simulink model "test_dc_motor_drive"  (R2025b)
settings: Solver=VariableStepAuto  StartTime=0.0  StopTime=8  RelTol=1e-3
StopFcn:
  | Simulink.sdi.view;
  | Simulink.sdi.loadView('view_dc_motor_drive.mldatx');
libraries: nesl_utility x5, fl_lib x4, ee_lib x1, arsenal x1, shareduavrstlib x1, simulink x1
settings Model: Creator=upattacini  LastModifiedBy=upattacini
settings SolverCC: DaesscMode=Robust  ZeroCrossAlgorithm=Adaptive  DecoupledContinuousIntegration=on  MinimalZcImpactIntegration=on
settings DataIOCC: SaveOutput=off  DSMLogging=off  SaveTime=off  ReturnWorkspaceOutputs=off

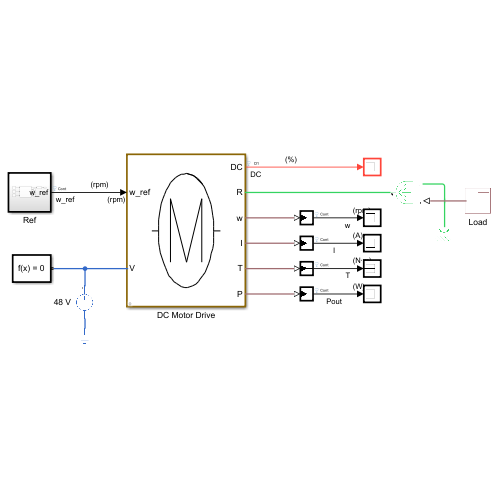
[thumbnail: Simulink's stored preview of the top-level diagram]
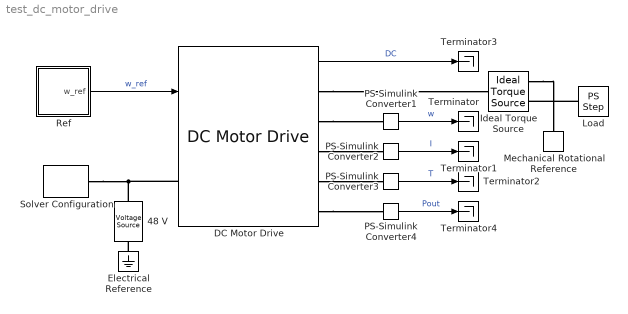
== system test_dc_motor_drive ==
  48 V : ee_lib/Sources/Voltage Source  dc_voltage=48 V  ac_voltage=0 V  ac_shift=0 rad  ac_frequency=60 Hz  noise_mode=ee.enum.sources.noise.Disabled  PSD=0 V^2/Hz  sample_time=1e-3 s  repeatability=ee.enum.sources.repeatability.NotRepeatable  user_seed=0  auto_seed=3499211588  i_specify=off  i_priority=None  i=0 A  i_nominal_specify=off  i_nominal_value=1  i_nominal_unit=A  v_specify=off  v_priority=None  v=0 V  v_nominal_specify=off  v_nominal_value=1  v_nominal_unit=V
  DC Motor Drive : arsenal/Simscape Components/Actuators/DC Motors/DC Motor Drive  R=0.58  L=0.0002  Kt=0.1564  T_bkpts=[0 0.774 1.564 2.71]  I_table=[0 4.95 10 17.325]  V_rated=48  GB_ratio=7.75  J=6.9927e-5  Kp=0.1  Ki=0.1  Ts=0.005  ff_bkpts=[0 60 120 180 240 310]  ff_table=[0 10 20 40 60 80]  V_max=100
  Electrical Reference : fl_lib/Electrical/Electrical Elements/Electrical Reference
  Ideal Torque Source : fl_lib/Mechanical/Mechanical Sources/Ideal Torque Source
  Load : fl_lib/Physical Signals/Sources/PS Step  step_time=4 s  initial_value=0 N*m  final_value=-1 N*m
  Mechanical Rotational Reference : fl_lib/Mechanical/Rotational Elements/Mechanical Rotational Reference
  PS-Simulink Converter1 : nesl_utility/PS-Simulink Converter  PhysicalDomain=network_engine_domain  SubClassName=ps_output  LeftPortType=input  RightPortType=output  PseudoPeriodic=off  Frequencies=[]  VectorFormat=inherit  Unit=rpm  AffineConversion=off
  PS-Simulink Converter2 : nesl_utility/PS-Simulink Converter  PhysicalDomain=network_engine_domain  SubClassName=ps_output  LeftPortType=input  RightPortType=output  PseudoPeriodic=off  Frequencies=[]  VectorFormat=inherit  Unit=A  AffineConversion=off
  PS-Simulink Converter3 : nesl_utility/PS-Simulink Converter  PhysicalDomain=network_engine_domain  SubClassName=ps_output  LeftPortType=input  RightPortType=output  PseudoPeriodic=off  Frequencies=[]  VectorFormat=inherit  Unit=N*m  AffineConversion=off
  PS-Simulink Converter4 : nesl_utility/PS-Simulink Converter  PhysicalDomain=network_engine_domain  SubClassName=ps_output  LeftPortType=input  RightPortType=output  PseudoPeriodic=off  Frequencies=[]  VectorFormat=inherit  Unit=W  AffineConversion=off
  Ref : Subsystem
  Solver Configuration : nesl_utility/Solver Configuration  PhysicalDomain=network_engine_domain  SubClassName=solver  LeftPortType=input  RightPortType=generic  Tones=[]  Harmonics=[]  SimulateNoise=off  Profile=off  UseLocalSampling=off  EnableSwitchedLinearOptims=on  FrequencyDomain=off  UseCCode=off  RelTol=0.001  AbsTol=0.001  MinStep=1e-09  ToWorkspace=off  RevertToSquareIcSolve=off  NumHomotopyIterations=100  PhasorMode=off  PhasorModeNumHarmonics=1  ConsistencySolver=NEWTON_XTOL_AFTER_FTOL  IndexReductionMethod=DerivativeReplacement  DoDC=off  ResidualTolerance=1e-09  ConsistencyTolSource=GLOBAL  ConsistencyAbsTol=0.001  ConsistencyRelTol=0.001  ConsistencyTolFactor=1  UseLocalSolver=off  LocalSolverChoice=NE_BACKWARD_EULER_ADVANCER  ResolveIndetEquations=on  FunctionEvalNumThread=1  LocalSolverSampleTime=0.001  DoFixedCost=off  MaxNonlinIter=3  MaxModeIter=2  ComputeImpulses=off  ImpulseIterations=2  LinearAlgebra=auto  LinearAlgebraNumThread=0  EquationFormulation=NE_TIME_EF  DelaysMemoryBudget=1024  AutomaticFiltering=on  FilteringTimeConstant=0.001  PartitionStorageMethod=AS_NEEDED  PartitionMemoryBudget=1024  PartitionMethod=ROBUST  MultibodyUseLocalSolver=off  MultibodyLocalSolverChoice=ODE1  MultibodyLocalSolverSampleTime=0.001
  Terminator{,1..4} (5 alike) : Terminator
  wires:
  Ref/1(w_ref) -> DC Motor Drive/1  "w_ref"
  PS-Simulink Converter2/1 -> Terminator1/1  "I"
  DC Motor Drive/1 -> Terminator3/1  "DC"
  PS-Simulink Converter1/1 -> Terminator/1  "w"
  PS-Simulink Converter3/1 -> Terminator2/1  "T"
  PS-Simulink Converter4/1 -> Terminator4/1  "Pout"
  connections:
  Electrical Reference/LConn1 -- 48 V/RConn1
  48 V/LConn1 -- Solver Configuration/RConn1 -- DC Motor Drive/LConn1
  DC Motor Drive/RConn3 -- PS-Simulink Converter2/LConn1
  DC Motor Drive/RConn2 -- PS-Simulink Converter1/LConn1
  DC Motor Drive/RConn4 -- PS-Simulink Converter3/LConn1
  Ideal Torque Source/RConn2 -- Mechanical Rotational Reference/LConn1
  Load/RConn1 -- Ideal Torque Source/RConn1
  DC Motor Drive/RConn1 -- Ideal Torque Source/LConn1
  DC Motor Drive/RConn5 -- PS-Simulink Converter4/LConn1

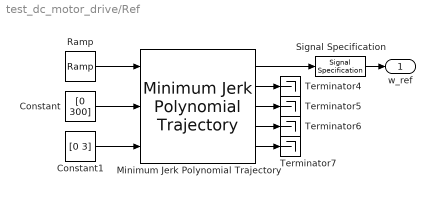
== system test_dc_motor_drive/Ref ==
  Constant : Constant  Value=[0 300]  VectorParams1D=off
  Constant1 : Constant  Value=[0 3]  VectorParams1D=off
  Minimum Jerk Polynomial Trajectory : shareduavrstlib/Minimum Jerk Polynomial Trajectory  ShowBCInputPort=off  ShowPolynomialCoefs=off  ShowStatusOutputPort=off  TimeAllocation=off  TimeWeight=100  MinSegmentTime=0.1  MaxSegmentTime=1  MaxIteration=1500  MaxTime=10  SimulateUsing=Interpreted execution
      settings: LibrarySourceBlock=robotutilslib/Minimum Jerk Polynomial Trajectory
  Ramp : simulink/Sources/Ramp  slope=1  start=0.3  InitialOutput=0
  Signal Specification : SignalSpecification  Unit=rpm
  Terminator{4..7} (4 alike) : Terminator
  w_ref : Outport
  wires:
  Minimum Jerk Polynomial Trajectory/3 -> Terminator5/1
  Constant/1 -> Minimum Jerk Polynomial Trajectory/2
  Constant1/1 -> Minimum Jerk Polynomial Trajectory/3
  Ramp/1 -> Minimum Jerk Polynomial Trajectory/1
  Minimum Jerk Polynomial Trajectory/4 -> Terminator6/1
  Minimum Jerk Polynomial Trajectory/2 -> Terminator4/1
  Minimum Jerk Polynomial Trajectory/5 -> Terminator7/1
  Minimum Jerk Polynomial Trajectory/1 -> Signal Specification/1
  Signal Specification/1 -> w_ref/1
